simulink model "PMSM_SIMULINK"  (R2022b)
settings: Solver=ode4  StartTime=0.0  StopTime=0.75  FixedStep=StepSize  RelTol=1e-3
values from neighbouring files (symbols this model uses):
  j = 100e-3    (= 0.1)    [PMSM_SCRIPT.m]
  ka = 0.3    [PMSM_SCRIPT.m]
  kf = 0.0008    [PMSM_SCRIPT.m]
  La = 2    [PMSM_SCRIPT.m]
  Ra = 1    [PMSM_SCRIPT.m]
  Ua = 30    [PMSM_SCRIPT.m]
settings Model: Creator=irfan  LastModifiedBy=irfan

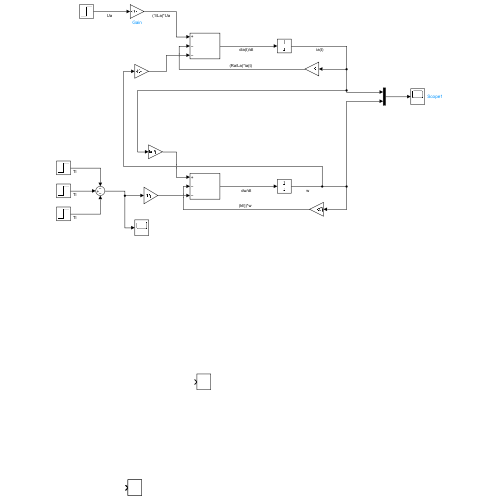
[thumbnail: Simulink's stored preview of the top-level diagram]
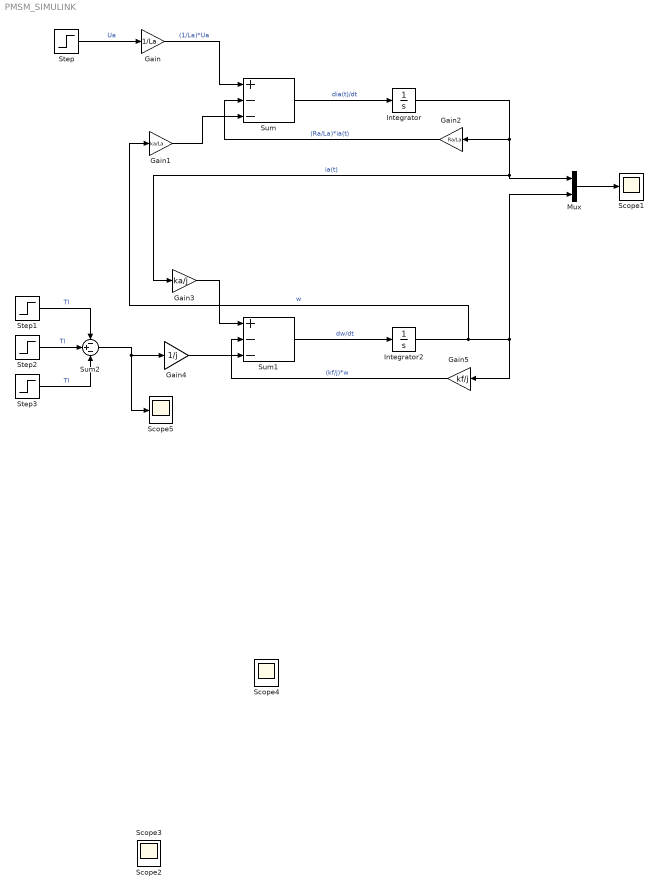
== system PMSM_SIMULINK ==
  Gain : Gain  Gain=1/La
  Gain1 : Gain  Gain=ka/La
  Gain2 : Gain  Gain=Ra/La
  Gain3 : Gain  Gain=ka/j
  Gain4 : Gain  Gain=1/j
  Gain5 : Gain  Gain=kf/j
  Integrator : Integrator
  Integrator2 : Integrator
  Mux : Mux  Inputs=2
  Scope{1..5} (5 alike) : Scope
  Step : Step  Time=0  Before=Ua  After=Ua  SampleTime=0
  Step1 : Step  Time=0  After=0.1  SampleTime=0
  Step2 : Step  Time=0.25  After=0.2  SampleTime=0
  Step3 : Step  Time=0.5  After=0.2  SampleTime=0
  Sum : Sum  Inputs=+--
  Sum1 : Sum  Inputs=+--
  Sum2 : Sum  Inputs=-+-
  wires:
  Integrator2/1 -> Gain1/1, Mux/2, Gain5/1  "w"
  Sum1/1 -> Integrator2/1  "dw/dt"
  Integrator/1 -> Gain3/1, Mux/1, Gain2/1  "ia(t)"
  Gain/1 -> Sum/1  "(1/La)*Ua"
  Gain3/1 -> Sum1/1
  Step/1 -> Gain/1  "Ua"
  Gain2/1 -> Sum/2  "(Ra/La)*ia(t)"
  Gain1/1 -> Sum/3
  Mux/1 -> Scope1/1
  Sum/1 -> Integrator/1  "dia(t)/dt"
  Gain5/1 -> Sum1/2  "(kf/j)*w"
  Gain4/1 -> Sum1/3
  Step1/1 -> Sum2/1  "Tl"
  Step2/1 -> Sum2/2  "Tl"
  Step3/1 -> Sum2/3  "Tl"
  Sum2/1 -> Scope5/1, Gain4/1
